simulink model "Modeling_Fix"  (R2023a)
settings: Solver=VariableStepAuto  StartTime=0.0  StopTime=40  RelTol=1e-3
undefined symbols (not defined in the file): ddx, ddy, ddz, dx, dy, dz, g, init, mass, ModelInit_AngEuler, ModelInit_PosE, ModelInit_RateB, ModelInit_VelB, ModelParam_uavJ, ModelParam_uavMass, p, pitch, q, r, roll, rotorCm, rotorCt, rotorD, ss_est_new, X, Y, yaw, Z
libraries: sharedutil x3, slident x1, slpidlib x1
settings Model: Creator=HP  LastModifiedBy=LENOVO

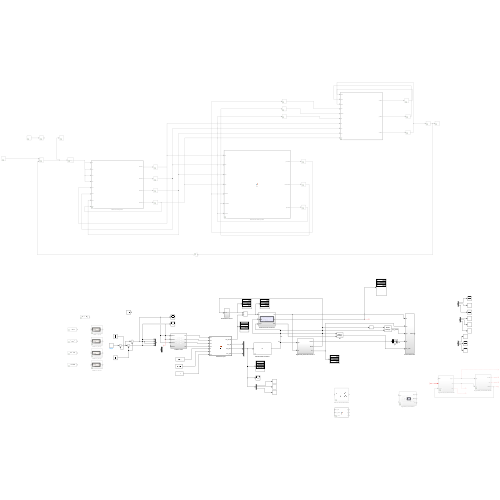
[thumbnail: Simulink's stored preview of the top-level diagram]
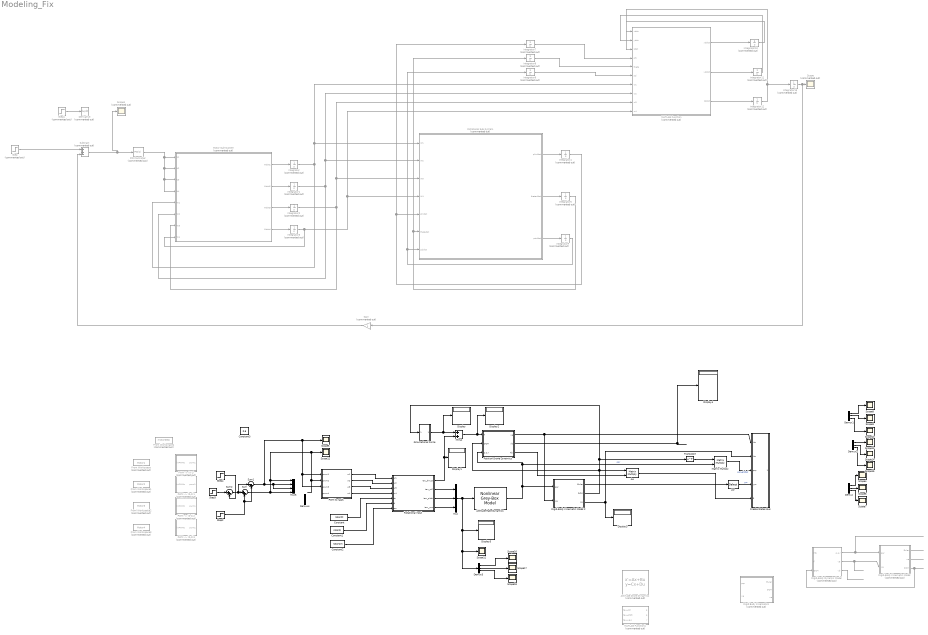
== system Modeling_Fix ==
  Ae : Product  Multiplication=Matrix(*)
  Attitude Drone Dynamics : StateSpace  Commented=on  A=ss_est_new.A  B=ss_est_new.B  C=ss_est_new.C  D=ss_est_new.D  InitialCondition=0
  Attitude Rate Dynamics : slident/Models/Nonlinear Grey-Box Model  nlsys=m  X0='m'
  Constant : Constant  Value=rotorCt
  Constant1 : Constant  Value=rotorD
  Constant2 : Constant  Value=rotorCm
  Constant3 : Constant  Value=0.6
  Create States Bus : Subsystem
  Demux{,1..3} (4 alike) : Demux  Outputs=3
  Demux4 : Demux
  Derivative : Derivative  Commented=on
  Display{,1..5} (6 alike) : Display
  From Workspace : FromWorkspace  Commented=on  VariableName=Motor1  SampleTime=0.25
  From Workspace1 : FromWorkspace  Commented=on  VariableName=Motor2  SampleTime=0.25
  From Workspace2 : FromWorkspace  Commented=on  VariableName=Motor3  SampleTime=0.25
  From Workspace3 : FromWorkspace  Commented=on  VariableName=Motor4  SampleTime=0.25
  From Workspace4 : FromWorkspace  Commented=on  VariableName=motorStep  SampleTime=0.25
  Gain : Gain  Commented=on
  Gravitational Force : Subsystem
  Integrator{,1..13} (14 alike) : Integrator  Commented=on
  MATLAB Function : MATLAB Function  Commented=on  TreatAsAtomicUnit=on
  MATLAB Function1 : MATLAB Function  Commented=on  TreatAsAtomicUnit=on
  Matrix Multiply : Product  Multiplication=Matrix(*)
  Minus : Sum
  Motor Sub-System : MATLAB Function  Commented=on  TreatAsAtomicUnit=on
  Mux : Mux  Inputs=3
  Mux5 : Mux
  PID Controller : slpidlib/PID Controller  Commented=on  Controller=PID  Form=Parallel  TimeDomain=Continuous-time  UseExternalTs=off  SampleTime=-1  IntegratorMethod=Forward Euler  FilterMethod=Forward Euler  ControllerParametersSource=internal  P=0.1  I=1  UseKiTs=off  D=0  N=100  UseFilter=on  TunerSelectOption=Transfer Function Based (PID Tuner App)  InitialConditionSource=internal  InitialConditionForIntegrator=0  InitialConditionForFilter=0  DifferentiatorICPrevScaledInput=0  ExternalReset=none  TrackingMode=off  Kt=1  LimitOutput=off  SatLimitsSource=internal  UpperSaturationLimit=inf  LowerSaturationLimit=-inf  LinearizeAsGain=on  AntiWindupMode=none  Kb=1  LimitIntegrator=off  UpperIntegratorSaturationLimit=inf  LowerIntegratorSaturationLimit=-inf  POutMin=[]  POutMax=[]  IOutMin=[]  IOutMax=[]  DOutMin=[]  DOutMax=[]  NOutMin=[]  NOutMax=[]  SumOutMin=[]  SumOutMax=[]  SaturationOutMin=[]  SaturationOutMax=[]  PParamMin=[]  PParamMax=[]  IParamMin=[]  IParamMax=[]  DParamMin=[]  DParamMax=[]  NParamMin=[]  NParamMax=[]  KbParamMin=[]  KbParamMax=[]  KtParamMin=[]  KtParamMax=[]  KbOutMin=[]  KbOutMax=[]  KtOutMin=[]  KtOutMax=[]  IntegratorOutMin=[]  IntegratorOutMax=[]  FilterOutMin=[]  FilterOutMax=[]  SumI1OutMin=[]  SumI1OutMax=[]  SumI2OutMin=[]  SumI2OutMax=[]  SumI3OutMin=[]  SumI3OutMax=[]  SumI4OutMin=[]  SumI4OutMax=[]  SumDOutMin=[]  SumDOutMax=[]  DifferentiatorOutMin=[]  DifferentiatorOutMax=[]  FilterDiffOutCoefMin=[]  FilterDiffOutCoefMax=[]  ReciprocalOutMin=[]  ReciprocalOutMax=[]  SumDenOutMin=[]  SumDenOutMax=[]  SumNumOutMin=[]  SumNumOutMax=[]  DivideOutMin=[]  DivideOutMax=[]  UdiffTsProdOutMin=[]  UdiffTsProdOutMax=[]  NTsProdOutMin=[]  NTsProdOutMax=[]  UintegralTsProdOutMin=[]  UintegralTsProdOutMax=[]  UngainTsProdOutMin=[]  UngainTsProdOutMax=[]  ClampingZeroOutDataTypeStr=Inherit: Inherit via back propagation  ClampingZeroOutMin=[]  ClampingZeroOutMax=[]  FilterDenConstantOutDataTypeStr=Inherit: Inherit via back propagation  FilterDenConstantOutMin=[]  FilterDenConstantOutMax=[]  PCopyOutDataTypeStr=Inherit: Inherit via back propagation  PCopyOutMin=[]  PCopyOutMax=[]  NCopyOutDataTypeStr=Inherit: Inherit via back propagation  NCopyOutMin=[]  NCopyOutMax=[]  IntegratorContinuousStateAttributes=''  IntegratorStateMustResolveToSignalObject=off  IntegratorRTWStateStorageClass=Auto  FilterContinuousStateAttributes=''  FilterStateMustResolveToSignalObject=off  FilterRTWStateStorageClass=Auto  ParallelPVariant=InternalParameters  IdealPVariant=Disabled  IVariant=InternalParameters  DVariant=InternalParameters  IntegratorVariant=Continuous  SatVariant=Disabled  AWVariant=Passthrough  PCopyVariant=Disabled  TRVariant=Disabled  FdbkBlocksVariant=Forward  IdealPFdbkVariant=Disabled  SatFdbkVariant=Disabled  DerivativeFilterVariant=ContFilter  NVariant=InternalParameters  NCopyVariant=Disabled  FilterICVariant=InternalICsFilter  IntegratorICVariant=InternalICs  ExternalResetVariant=Disabled  TRSumVariant=Passthrough  SumFdbkVariant=Disabled  SumVariant=Sum_PID  TsampFilterVariant=InternalTs  TsampNgainVariant=Passthrough  TsampIntegralVariant=Disabled_SignalSpec  ExternalSaturationOutDataTypeStr=Inherit: Same as second input
  "PWM -> (0-1)" : Subsystem  Commented=on
  "PWM -> (0-1)1" : Subsystem  Commented=on
  "PWM -> (0-1)2" : Subsystem  Commented=on
  "PWM -> (0-1)3" : Subsystem  Commented=on
  PWM to rad/s : Subsystem
  Position Drone Dynamics : Subsystem
  Rigid Body Kinematics : Subsystem  Commented=on
  Rigid-Body Dynamic Model : Subsystem  Commented=on
  "Rigid-Body Kinematic Model " : Subsystem  Commented=on
  Rigid-Body Kinematic Model 2 : Subsystem
  Rotational Input : MATLAB Function  TreatAsAtomicUnit=on
  Rotational Sub-System : MATLAB Function  Commented=on  TreatAsAtomicUnit=on
  Scope : Scope  Commented=on
  Scope1 : Scope  Commented=on
  Scope{4..18} (15 alike) : Scope
  Step : Step  Commented=on  Time=0  SampleTime=0
  Step1 : Step  Commented=on  Time=200  After=99  SampleTime=0
  Step2 : Step  Time=0  After=0.9  SampleTime=0.25
  Step3 : Step  Time=10  After=0.01  SampleTime=0.25
  Step4 : Step  Time=11  After=0.01  SampleTime=0.25
  Subtract : Sum  Commented=on  Inputs=++-
  Sum : Sum  Inputs=|++
  Sum1 : Sum  Inputs=|-+
  Sum2 : Sum  Inputs=|+-
  Transpose : Math  Operator=transpose
  ypr : Selector  InputPortWidth=3  IndexOptions=Index vector (dialog)  Indices=[3 2 1]  OutputSizes=1
  wires:
  Motor Sub-System/1(Wdot1) -> Integrator/1
  Integrator/1 -> MATLAB Function/7(w1), Rotational Sub-System/1(W1), Motor Sub-System/5(W1)
  Motor Sub-System/2(Wdot2) -> Integrator1/1
  Motor Sub-System/3(Wdot3) -> Integrator2/1
  Motor Sub-System/4(Wdot4) -> Integrator3/1
  Integrator1/1 -> MATLAB Function/8(w2), Rotational Sub-System/2(W2), Motor Sub-System/6(W2)
  Integrator2/1 -> MATLAB Function/9(w3), Rotational Sub-System/3(W3), Motor Sub-System/7(W3)
  Integrator3/1 -> MATLAB Function/10(w4), Rotational Sub-System/4(W4), Motor Sub-System/8(W4)
  Rotational Sub-System/1(phiddot) -> Integrator4/1
  Integrator4/1 -> Integrator7/1, Rotational Sub-System/5(phidot)
  Rotational Sub-System/2(thetaddot) -> Integrator5/1
  Integrator5/1 -> Integrator8/1, Rotational Sub-System/6(thetadot)
  Rotational Sub-System/3(psiddot) -> Integrator6/1
  Integrator6/1 -> Integrator9/1, Rotational Sub-System/7(psidot)
  Integrator7/1 -> MATLAB Function/4(phi)
  Integrator8/1 -> MATLAB Function/5(theta)
  Integrator9/1 -> MATLAB Function/6(psi)
  MATLAB Function/1(xddot) -> Integrator10/1
  Integrator10/1 -> MATLAB Function/1(xdot)
  MATLAB Function/2(yddot) -> Integrator11/1
  Integrator11/1 -> MATLAB Function/2(ydot)
  Integrator12/1 -> MATLAB Function/3(zdot), Integrator13/1
  MATLAB Function/3(zddot) -> Integrator12/1
  Step/1 -> Subtract/1
  Gain/1 -> Subtract/3
  Integrator13/1 -> Gain/1, Scope/1
  Subtract/1 -> PID Controller/1, Scope1/1
  Step1/1 -> Derivative/1
  PID Controller/1 -> Motor Sub-System/4(U4), Motor Sub-System/3(U3), Motor Sub-System/2(U2), Motor Sub-System/1(U1)
  PWM to rad/s/1(w1) -> Rotational Input/1(w1)
  PWM to rad/s/2(w2) -> Rotational Input/2(w2)
  PWM to rad/s/3(w3) -> Rotational Input/3(w3)
  PWM to rad/s/4(w4) -> Rotational Input/4(w4)
  Mux/1 -> Scope11/1, Demux3/1, Display5/1, Attitude Rate Dynamics/1
  Rotational Input/1(tau_thrust) -> Minus/2, Display1/1
  Attitude Rate Dynamics/1 -> Position Drone Dynamics/3(p,q,r), Matrix Multiply/2, Rigid-Body Kinematic Model 2/1(pqr)  "pqr"
  "Rigid-Body Kinematic Model "/3(DCM) -> Rigid-Body Dynamic Model/3(DCM)
  ? -> Rigid-Body Dynamic Model/2(f)
  Rigid-Body Dynamic Model/1("p,q,r ") -> "Rigid-Body Kinematic Model "/1(pqr)
  "Rigid-Body Kinematic Model "/2("xe ") -> ?
  Rigid-Body Dynamic Model/3("vb ") -> ?
  Rigid-Body Dynamic Model/2(ve) -> "Rigid-Body Kinematic Model "/2(ve)
  "Rigid-Body Kinematic Model "/1(Euler) -> ?
  Rotational Input/2(tau_roll) -> Mux/1
  Rotational Input/3(tau_pitch) -> Mux/2
  Rotational Input/4(tau_yaw) -> Mux/3
  Rigid-Body Kinematic Model 2/1(Euler) -> ypr/1
  Position Drone Dynamics/1(ve) -> Rigid-Body Kinematic Model 2/2(ve), Create States Bus/1(Ve)
  Position Drone Dynamics/2(vb) -> Display4/1
  Position Drone Dynamics/3(Ab) -> Ae/2
  Ae/1 -> Create States Bus/5(acc_lnav)
  Constant/1 -> Rotational Input/5(ct)
  Constant1/1 -> Rotational Input/6(d)
  Constant2/1 -> Rotational Input/7(cm)
  Rigid-Body Kinematic Model 2/2(DCM) -> Transpose/1, Gravitational Force/1(DCM), Position Drone Dynamics/2(DCM), Ae/1
  Gravitational Force/1(Out1) -> Display/1, Minus/1
  Minus/1 -> Display2/1, Position Drone Dynamics/1(f)
  Step4/1 -> Sum2/2
  Step3/1 -> Sum2/1
  Step2/1 -> Sum1/2, Sum/2
  Sum/1 -> PWM to rad/s/2(pwm2), Scope12/1, Mux5/1, Mux5/4
  Sum2/1 -> Sum1/1, Sum/1
  Demux/1 -> Scope4/1
  Demux/2 -> Scope6/1
  Demux/3 -> Scope7/1
  Demux1/2 -> Scope9/1
  Demux1/3 -> Scope10/1
  Demux1/1 -> Scope8/1
  Sum1/1 -> PWM to rad/s/3(pwm3), PWM to rad/s/1(pwm1), Scope5/1, Mux5/2, Mux5/3
  Demux2/1 -> Scope13/1
  Demux2/2 -> Scope14/1
  Demux2/3 -> Scope15/1
  Demux3/2 -> Scope17/1
  Demux3/1 -> Scope16/1
  Demux3/3 -> Scope18/1
  Rigid-Body Kinematic Model 2/3("xe ") -> Create States Bus/2(Xe), Display3/1
  ypr/1 -> Create States Bus/4(ypr)  "ypr"
  Transpose/1 -> Matrix Multiply/1
  Matrix Multiply/1 -> Create States Bus/3(pqr)  "pqr_global"

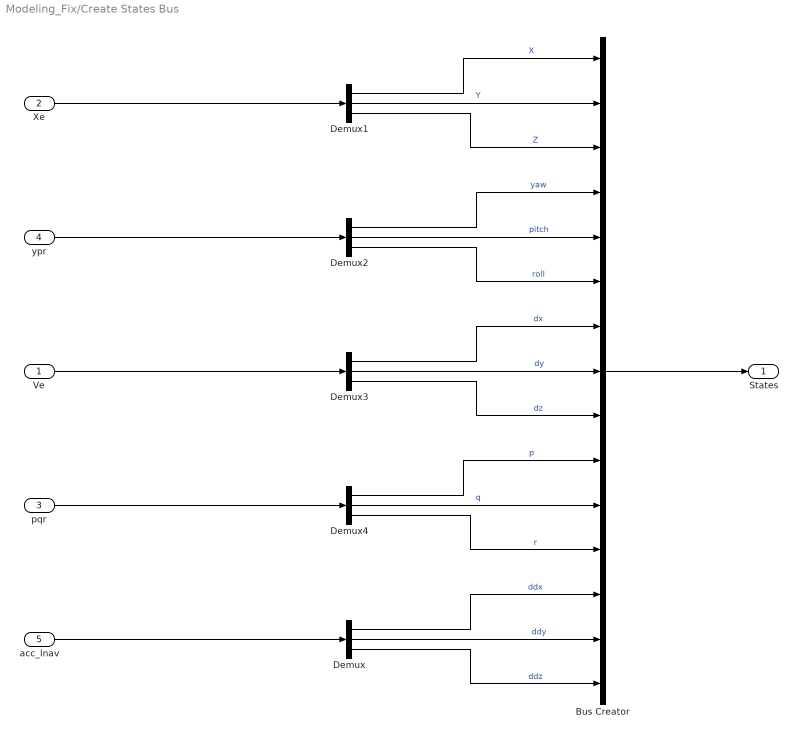
== system Modeling_Fix/Create States Bus ==
  Ve : Inport
  Xe : Inport  Port=2
  pqr : Inport  Port=3
  ypr : Inport  Port=4
  acc_lnav : Inport  Port=5
  Bus Creator : BusCreator  Inputs=X,Y,Z,yaw,pitch,roll,dx,dy,dz,p,q,r,ddx,ddy,ddz
  Demux{,1..4} (5 alike) : Demux  Outputs=3
  States : Outport
  wires:
  Demux1/1 -> Bus Creator/1  "X"
  Demux1/2 -> Bus Creator/2  "Y"
  ypr/1 -> Demux2/1
  Demux2/2 -> Bus Creator/5  "pitch"
  Demux3/2 -> Bus Creator/8  "dy"
  Demux2/3 -> Bus Creator/6  "roll"
  pqr/1 -> Demux4/1
  Ve/1 -> Demux3/1
  Demux2/1 -> Bus Creator/4  "yaw"
  Demux1/3 -> Bus Creator/3  "Z"
  Demux3/1 -> Bus Creator/7  "dx"
  Demux4/2 -> Bus Creator/11  "q"
  Demux3/3 -> Bus Creator/9  "dz"
  Demux4/3 -> Bus Creator/12  "r"
  Demux4/1 -> Bus Creator/10  "p"
  Bus Creator/1 -> States/1
  Xe/1 -> Demux1/1
  acc_lnav/1 -> Demux/1
  Demux/3 -> Bus Creator/15  "ddz"
  Demux/2 -> Bus Creator/14  "ddy"
  Demux/1 -> Bus Creator/13  "ddx"

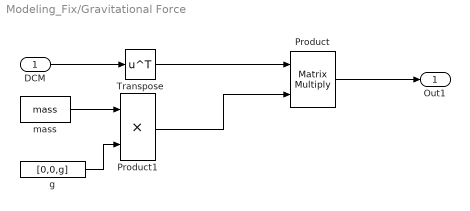
== system Modeling_Fix/Gravitational Force ==
  DCM : Inport
  Product : Product  Multiplication=Matrix(*)
  Product1 : Product
  Transpose : Math  Operator=transpose  SignedPower=on
  g : Constant  Value=[0,0,g]
  mass : Constant  Value=mass
  Out1 : Outport
  wires:
  Transpose/1 -> Product/1
  Product/1 -> Out1/1
  g/1 -> Product1/2
  mass/1 -> Product1/1
  Product1/1 -> Product/2
  DCM/1 -> Transpose/1

== system Modeling_Fix/PWM -> (0-1) ==
  note: The input is a PWM signal from 1000 to 2000,
      | which needs to be normalized to 0~1.
  inPWMs : Inport
  Constant2 : Constant  Value=900
  Gain1 : Gain  Gain=1/1100
  Saturation : Saturate  UpperLimit=1  LowerLimit=0
  Sum : Sum  Inputs=|+-
  pwm1 : Outport
  wires:
  inPWMs/1 -> Sum/1
  Constant2/1 -> Sum/2
  Gain1/1 -> Saturation/1
  Sum/1 -> Gain1/1
  Saturation/1 -> pwm1/1

== system Modeling_Fix/PWM -> (0-1)1 ==
  note: The input is a PWM signal from 1000 to 2000,
      | which needs to be normalized to 0~1.
  inPWMs : Inport
  Constant2 : Constant  Value=900
  Gain1 : Gain  Gain=1/1100
  Saturation : Saturate  UpperLimit=1  LowerLimit=0
  Sum : Sum  Inputs=|+-
  pwm1 : Outport
  wires:
  inPWMs/1 -> Sum/1
  Constant2/1 -> Sum/2
  Gain1/1 -> Saturation/1
  Sum/1 -> Gain1/1
  Saturation/1 -> pwm1/1

== system Modeling_Fix/PWM -> (0-1)2 ==
  note: The input is a PWM signal from 1000 to 2000,
      | which needs to be normalized to 0~1.
  inPWMs : Inport
  Constant2 : Constant  Value=900
  Gain1 : Gain  Gain=1/1100
  Saturation : Saturate  UpperLimit=1  LowerLimit=0
  Sum : Sum  Inputs=|+-
  pwm1 : Outport
  wires:
  inPWMs/1 -> Sum/1
  Constant2/1 -> Sum/2
  Gain1/1 -> Saturation/1
  Sum/1 -> Gain1/1
  Saturation/1 -> pwm1/1

== system Modeling_Fix/PWM -> (0-1)3 ==
  note: The input is a PWM signal from 1000 to 2000,
      | which needs to be normalized to 0~1.
  inPWMs : Inport
  Constant2 : Constant  Value=900
  Gain1 : Gain  Gain=1/1100
  Saturation : Saturate  UpperLimit=1  LowerLimit=0
  Sum : Sum  Inputs=|+-
  pwm1 : Outport
  wires:
  inPWMs/1 -> Sum/1
  Constant2/1 -> Sum/2
  Gain1/1 -> Saturation/1
  Sum/1 -> Gain1/1
  Saturation/1 -> pwm1/1

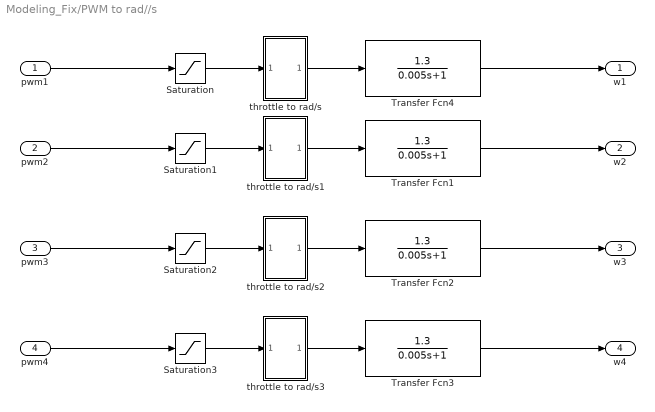
== system Modeling_Fix/PWM to rad//s ==
  pwm1 : Inport
  pwm2 : Inport  Port=2
  pwm3 : Inport  Port=3
  pwm4 : Inport  Port=4
  Saturation{,1..3} (4 alike) : Saturate  UpperLimit=1  LowerLimit=0
  Transfer Fcn{1..4} (4 alike) : TransferFcn  Numerator=1.3  Denominator=[0.005 1]
  throttle to rad/s : Subsystem
  throttle to rad/s1 : Subsystem
  throttle to rad/s2 : Subsystem
  throttle to rad/s3 : Subsystem
  w1 : Outport
  w2 : Outport  Port=2
  w3 : Outport  Port=3
  w4 : Outport  Port=4
  wires:
  pwm1/1 -> Saturation/1
  pwm2/1 -> Saturation1/1
  throttle to rad/s/1(Out1) -> Transfer Fcn4/1
  Transfer Fcn4/1 -> w1/1
  throttle to rad/s3/1(Out1) -> Transfer Fcn3/1
  Transfer Fcn1/1 -> w2/1
  throttle to rad/s2/1(Out1) -> Transfer Fcn2/1
  Transfer Fcn3/1 -> w4/1
  pwm4/1 -> Saturation3/1
  Transfer Fcn2/1 -> w3/1
  pwm3/1 -> Saturation2/1
  Saturation/1 -> throttle to rad/s/1(In2)
  Saturation1/1 -> throttle to rad/s1/1(In2)
  Saturation2/1 -> throttle to rad/s2/1(In2)
  Saturation3/1 -> throttle to rad/s3/1(In2)
  throttle to rad/s1/1(Out1) -> Transfer Fcn1/1

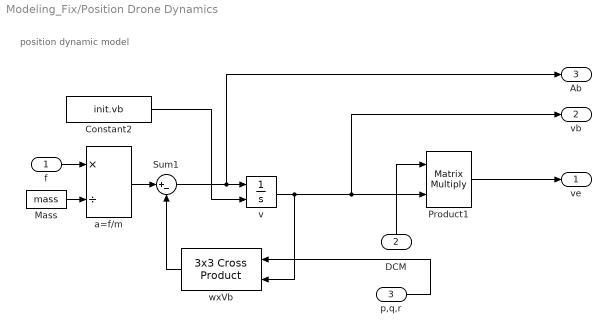
== system Modeling_Fix/Position Drone Dynamics ==
  note: position dynamic model
  f : Inport
  DCM : Inport  Port=2
  p,q,r : Inport  Port=3
  " Mass " : Constant  Value=mass
  Constant2 : Constant  Value=init.vb
  Product1 : Product  Multiplication=Matrix(*)
  Sum1 : Sum  Inputs=|+-
  a=f/m : Product  Inputs=*/
  v : Integrator  InitialConditionSource=external
  wxVb : sharedutil/3x3 Cross Product  aMode=aMode
  ve : Outport  VectorParamsAs1DForOutWhenUnconnected=off
  vb : Outport  Port=2  VectorParamsAs1DForOutWhenUnconnected=off
  Ab : Outport  Port=3
  wires:
  DCM/1 -> Product1/1
  v/1 -> vb/1, Product1/2, wxVb/2
  Sum1/1 -> Ab/1, v/1
  Constant2/1 -> v/2
  " Mass "/1 -> a=f/m/2
  wxVb/1 -> Sum1/2
  f/1 -> a=f/m/1
  p,q,r/1 -> wxVb/1
  a=f/m/1 -> Sum1/1
  Product1/1 -> ve/1

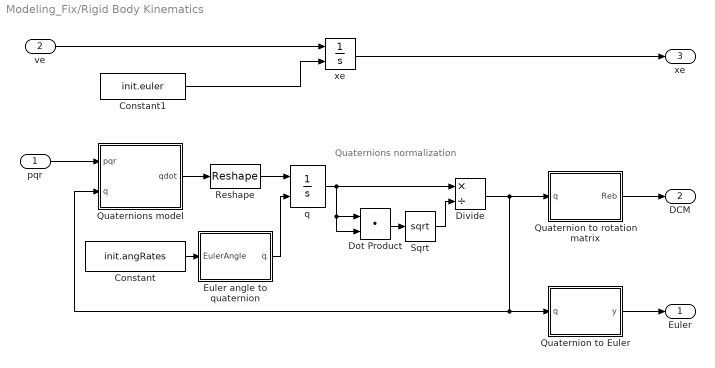
== system Modeling_Fix/Rigid Body Kinematics ==
  note: Quaternions
      | normalization
  pqr : Inport
  ve : Inport  Port=2
  Constant : Constant  Value=init.angRates
  Constant1 : Constant  Value=init.euler
  Divide : Product  Inputs=*/
  Dot Product : DotProduct  OutDataTypeStr=Inherit: Inherit via internal rule
  Euler angle to quaternion : MATLAB Function
  Quaternion to Euler : MATLAB Function
  Quaternion to rotation matrix : MATLAB Function
  Quaternions model : MATLAB Function  TreatAsAtomicUnit=on
  Reshape : Reshape  OutputDimensionality=Customize  OutputDimensions=[4,1]
  Sqrt : Sqrt
  q : Integrator  InitialConditionSource=external
  xe : Integrator  InitialConditionSource=external
  Euler : Outport  VectorParamsAs1DForOutWhenUnconnected=off
  DCM : Outport  Port=2  VectorParamsAs1DForOutWhenUnconnected=off
  "xe " : Outport  Port=3  VectorParamsAs1DForOutWhenUnconnected=off
  wires:
  q/1 -> Divide/1, Dot Product/1, Dot Product/2
  Quaternion to Euler/1(y) -> Euler/1
  Divide/1 -> Quaternion to rotation matrix/1(q), Quaternions model/2(q), Quaternion to Euler/1(q)
  Reshape/1 -> q/1
  Dot Product/1 -> Sqrt/1
  Sqrt/1 -> Divide/2
  pqr/1 -> Quaternions model/1(pqr)
  Euler angle to quaternion/1(q) -> q/2
  Quaternions model/1(qdot) -> Reshape/1
  Constant/1 -> Euler angle to quaternion/1(EulerAngle)
  Quaternion to rotation matrix/1(Reb) -> DCM/1
  Constant1/1 -> xe/2
  ve/1 -> xe/1
  xe/1 -> "xe "/1

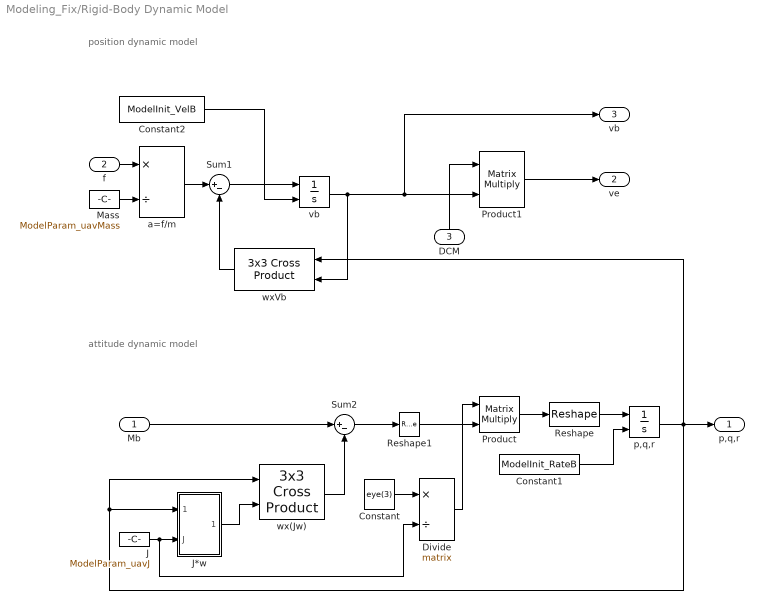
== system Modeling_Fix/Rigid-Body Dynamic Model ==
  note: attitude dynamic model
  note: position dynamic model
  Mb : Inport
  f : Inport  Port=2
  DCM : Inport  Port=3
  " Mass " : Constant  Value=ModelParam_uavMass
  Constant : Constant  Value=eye(3)
  Constant1 : Constant  Value=ModelInit_RateB
  Constant2 : Constant  Value=ModelInit_VelB
  Divide : Product  Inputs=*/  Multiplication=Matrix(*)
  "J " : Constant  Value=ModelParam_uavJ
  J*w : Subsystem
  Product : Product  Multiplication=Matrix(*)
  Product1 : Product  Multiplication=Matrix(*)
  Reshape : Reshape  OutputDimensionality=Customize  OutputDimensions=[3,1]
  Reshape1 : Reshape  OutputDimensionality=Column vector (2-D)
  Sum1 : Sum  Inputs=|+-
  Sum2 : Sum  Inputs=|+-
  a=f/m : Product  Inputs=*/
  p,q,r : Integrator  InitialConditionSource=external
  vb : Integrator  InitialConditionSource=external
  wx(Jw) : sharedutil/3x3 Cross Product  aMode=aMode
  wxVb : sharedutil/3x3 Cross Product  aMode=aMode
  "p,q,r " : Outport  VectorParamsAs1DForOutWhenUnconnected=off
  ve : Outport  Port=2  VectorParamsAs1DForOutWhenUnconnected=off
  "vb " : Outport  Port=3  VectorParamsAs1DForOutWhenUnconnected=off
  wires:
  Product/1 -> Reshape/1
  Reshape1/1 -> Product/2
  Constant/1 -> Divide/1
  Divide/1 -> Product/1
  Sum2/1 -> Reshape1/1
  "J "/1 -> Divide/2, J*w/2(J)
  p,q,r/1 -> "p,q,r "/1, J*w/1(p q r), wx(Jw)/1, wxVb/1
  J*w/1("J*w ") -> wx(Jw)/2
  Mb/1 -> Sum2/1
  wx(Jw)/1 -> Sum2/2
  Constant2/1 -> vb/2
  f/1 -> a=f/m/1
  Product1/1 -> ve/1
  wxVb/1 -> Sum1/2
  a=f/m/1 -> Sum1/1
  Sum1/1 -> vb/1
  vb/1 -> Product1/2, "vb "/1, wxVb/2
  " Mass "/1 -> a=f/m/2
  DCM/1 -> Product1/1
  Reshape/1 -> p,q,r/1
  Constant1/1 -> p,q,r/2

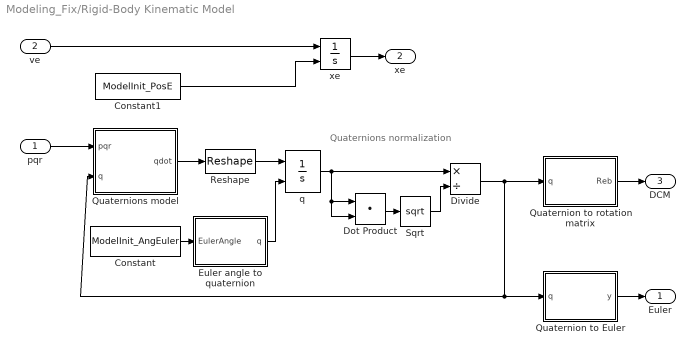
== system Modeling_Fix/Rigid-Body Kinematic Model  ==
  note: Quaternions
      | normalization
  pqr : Inport
  ve : Inport  Port=2
  Constant : Constant  Value=ModelInit_AngEuler
  Constant1 : Constant  Value=ModelInit_PosE
  Divide : Product  Inputs=*/
  Dot Product : DotProduct  OutDataTypeStr=Inherit: Inherit via internal rule
  Euler angle to quaternion : MATLAB Function
  Quaternion to Euler : MATLAB Function
  Quaternion to rotation matrix : MATLAB Function
  Quaternions model : MATLAB Function  TreatAsAtomicUnit=on
  Reshape : Reshape  OutputDimensionality=Customize  OutputDimensions=[4,1]
  Sqrt : Sqrt
  q : Integrator  InitialConditionSource=external
  xe : Integrator  InitialConditionSource=external
  Euler : Outport  VectorParamsAs1DForOutWhenUnconnected=off
  "xe " : Outport  Port=2  VectorParamsAs1DForOutWhenUnconnected=off
  DCM : Outport  Port=3  VectorParamsAs1DForOutWhenUnconnected=off
  wires:
  Divide/1 -> Quaternion to rotation matrix/1(q), Quaternions model/2(q), Quaternion to Euler/1(q)
  Dot Product/1 -> Sqrt/1
  pqr/1 -> Quaternions model/1(pqr)
  q/1 -> Divide/1, Dot Product/1, Dot Product/2
  Quaternions model/1(qdot) -> Reshape/1
  Quaternion to rotation matrix/1(Reb) -> DCM/1
  Quaternion to Euler/1(y) -> Euler/1
  Constant/1 -> Euler angle to quaternion/1(EulerAngle)
  Euler angle to quaternion/1(q) -> q/2
  Reshape/1 -> q/1
  ve/1 -> xe/1
  xe/1 -> "xe "/1
  Constant1/1 -> xe/2
  Sqrt/1 -> Divide/2

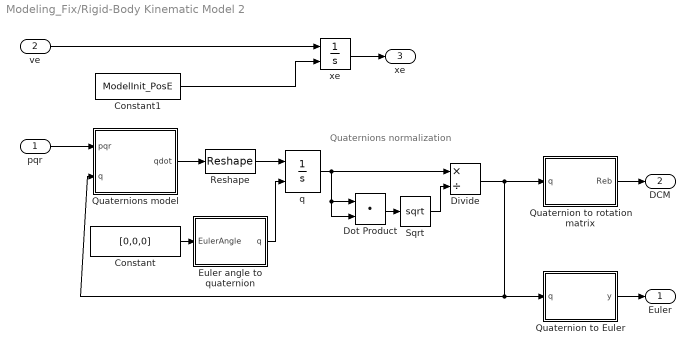
== system Modeling_Fix/Rigid-Body Kinematic Model 2 ==
  note: Quaternions
      | normalization
  pqr : Inport
  ve : Inport  Port=2
  Constant : Constant  Value=[0,0,0]
  Constant1 : Constant  Value=ModelInit_PosE
  Divide : Product  Inputs=*/
  Dot Product : DotProduct  OutDataTypeStr=Inherit: Inherit via internal rule
  Euler angle to quaternion : MATLAB Function
  Quaternion to Euler : MATLAB Function
  Quaternion to rotation matrix : MATLAB Function
  Quaternions model : MATLAB Function  TreatAsAtomicUnit=on
  Reshape : Reshape  OutputDimensionality=Customize  OutputDimensions=[4,1]
  Sqrt : Sqrt
  q : Integrator  InitialConditionSource=external
  xe : Integrator  InitialConditionSource=external
  Euler : Outport  VectorParamsAs1DForOutWhenUnconnected=off
  DCM : Outport  Port=2  VectorParamsAs1DForOutWhenUnconnected=off
  "xe " : Outport  Port=3  VectorParamsAs1DForOutWhenUnconnected=off
  wires:
  Divide/1 -> Quaternion to rotation matrix/1(q), Quaternions model/2(q), Quaternion to Euler/1(q)
  Dot Product/1 -> Sqrt/1
  pqr/1 -> Quaternions model/1(pqr)
  q/1 -> Divide/1, Dot Product/1, Dot Product/2
  Quaternions model/1(qdot) -> Reshape/1
  Quaternion to rotation matrix/1(Reb) -> DCM/1
  Quaternion to Euler/1(y) -> Euler/1
  Constant/1 -> Euler angle to quaternion/1(EulerAngle)
  Euler angle to quaternion/1(q) -> q/2
  Reshape/1 -> q/1
  ve/1 -> xe/1
  xe/1 -> "xe "/1
  Constant1/1 -> xe/2
  Sqrt/1 -> Divide/2

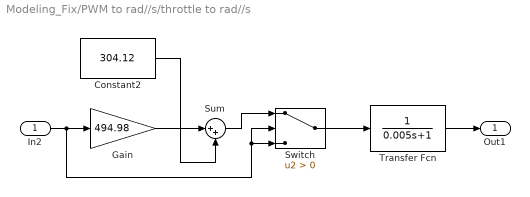
== system Modeling_Fix/PWM to rad//s/throttle to rad//s ==
  In2 : Inport
  Constant2 : Constant  Value=304.12
  Gain : Gain  Gain=494.98
  Sum : Sum  Inputs=|++
  Switch : Switch  Criteria=u2 > Threshold  SaturateOnIntegerOverflow=off  InputSameDT=off
  Transfer Fcn : TransferFcn  Denominator=[0.005 1]
  Out1 : Outport
  wires:
  Constant2/1 -> Sum/2
  Gain/1 -> Sum/1
  In2/1 -> Switch/3, Switch/2, Gain/1
  Sum/1 -> Switch/1
  Transfer Fcn/1 -> Out1/1
  Switch/1 -> Transfer Fcn/1

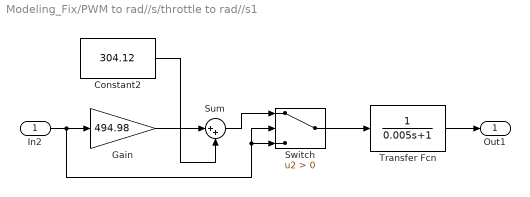
== system Modeling_Fix/PWM to rad//s/throttle to rad//s1 ==
  In2 : Inport
  Constant2 : Constant  Value=304.12
  Gain : Gain  Gain=494.98
  Sum : Sum  Inputs=|++
  Switch : Switch  Criteria=u2 > Threshold  SaturateOnIntegerOverflow=off  InputSameDT=off
  Transfer Fcn : TransferFcn  Denominator=[0.005 1]
  Out1 : Outport
  wires:
  Constant2/1 -> Sum/2
  Gain/1 -> Sum/1
  In2/1 -> Switch/3, Switch/2, Gain/1
  Sum/1 -> Switch/1
  Transfer Fcn/1 -> Out1/1
  Switch/1 -> Transfer Fcn/1

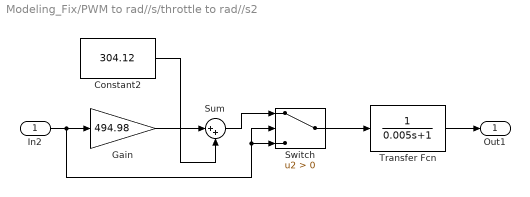
== system Modeling_Fix/PWM to rad//s/throttle to rad//s2 ==
  In2 : Inport
  Constant2 : Constant  Value=304.12
  Gain : Gain  Gain=494.98
  Sum : Sum  Inputs=|++
  Switch : Switch  Criteria=u2 > Threshold  SaturateOnIntegerOverflow=off  InputSameDT=off
  Transfer Fcn : TransferFcn  Denominator=[0.005 1]
  Out1 : Outport
  wires:
  Constant2/1 -> Sum/2
  Gain/1 -> Sum/1
  In2/1 -> Switch/3, Switch/2, Gain/1
  Sum/1 -> Switch/1
  Transfer Fcn/1 -> Out1/1
  Switch/1 -> Transfer Fcn/1

== system Modeling_Fix/PWM to rad//s/throttle to rad//s3 ==
  In2 : Inport
  Constant2 : Constant  Value=304.12
  Gain : Gain  Gain=494.98
  Sum : Sum  Inputs=|++
  Switch : Switch  Criteria=u2 > Threshold  SaturateOnIntegerOverflow=off  InputSameDT=off
  Transfer Fcn : TransferFcn  Denominator=[0.005 1]
  Out1 : Outport
  wires:
  Constant2/1 -> Sum/2
  Gain/1 -> Sum/1
  In2/1 -> Switch/3, Switch/2, Gain/1
  Sum/1 -> Switch/1
  Transfer Fcn/1 -> Out1/1
  Switch/1 -> Transfer Fcn/1

== system Modeling_Fix/Rigid-Body Dynamic Model/J*w ==
  p q r : Inport
  J : Inport  Port=2
  J*w : Product  Multiplication=Matrix(*)
  "J*w " : Outport  VectorParamsAs1DForOutWhenUnconnected=off
  wires:
  J*w/1 -> "J*w "/1
  J/1 -> J*w/1
  p q r/1 -> J*w/2

== matlab function Modeling_Fix/Rigid-Body Kinematic Model /Quaternion to rotation matrix ==
  data: q input; Reb output
function Reb = fcn(q)
%Function description;
%  The rotation matrix of the Aircraft-Body Coordinate Frame (ABCF) to the
%  Earth-Fixed Coordinate Frame (EFCF) is obtained from the quaternions
Reb = [q(1)*q(1) + q(2)*q(2) - q(3)*q(3) - q(4)*q(4), 2*(q(2)*q(3) - q(1)*q(4)), 2*(q(2)*q(4) + q(1)*q(3))
           2*(q(2)*q(3) + q(1)*q(4)), q(1)*q(1) - q(2)*q(2) + q(3)*q(3) - q(4)*q(4), 2*(q(3)*q(4) - q(1)*q(2))
           2*(q(2)*q(4) - q(1)*q(3)), 2*(q(3)*q(4) + q(1)*q(2)), q(1)*q(1) - q(2)*q(2) - q(3)*q(3) + q(4)*q(4)];

== matlab function Modeling_Fix/Rigid-Body Kinematic Model /Quaternion to Euler ==
  data: q input; y output
function y = fcn(q)
 %Function description:
%  Quaternions to Euler
phi = atan2(2*(q(1)*q(2) + q(3)*q(4)), (1 - 2*(q(2)*q(2) + q(3)*q(3))));
theta = asin(2*(q(1)*q(3) - q(2)*q(4)));
psi = atan2(2*(q(1)*q(4) + q(2)*q(3)), (1 - 2*(q(3)*q(3) + q(4)*q(4))));
y = [phi theta psi];

== matlab function Modeling_Fix/Rigid-Body Kinematic Model /Quaternions model ==
  data: pqr input; qdot output; q input
function qdot = fcn(pqr, q)
%Function description:
%  Quaternions model
qdot = 0.5*[0, -pqr(1), -pqr(2), -pqr(3); pqr(1), 0, pqr(3), -pqr(2); pqr(2), -pqr(3), 0, pqr(1); pqr(3), pqr(2), -pqr(1), 0]*q;

== matlab function Modeling_Fix/Rigid-Body Kinematic Model /Euler angle to quaternion ==
  data: EulerAngle input; q output
function q = fcn(EulerAngle)
%Function description:
%  Get quaternions from Euler angle
q0 =  cos(EulerAngle(1)/2)*cos(EulerAngle(2)/2)*cos(EulerAngle(3)/2) + sin(EulerAngle(1)/2)*sin((EulerAngle(2)/2))*sin((EulerAngle(3)/2));
q1 = sin(EulerAngle(1)/2)*cos(EulerAngle(2)/2)*cos(EulerAngle(3)/2) - cos(EulerAngle(1)/2)*sin((EulerAngle(2)/2))*sin((EulerAngle(3)/2));
q2 = cos(EulerAngle(1)/2)*sin(EulerAngle(2)/2)*cos(EulerAngle(3)/2) + sin(EulerAngle(1)/2)*cos((EulerAngle(2)/2))*sin((EulerAngle(3)/2));
q3 = cos(EulerAngle(1)/2)*cos(EulerAngle(2)/2)*sin(EulerAngle(3)/2) - sin(EulerAngle(1)/2)*sin((EulerAngle(2)/2))*cos((EulerAngle(3)/2));
q = [q0 q1 q2 q3]';

== matlab function Modeling_Fix/Rigid Body Kinematics/Quaternion to Euler ==
  data: q input; y output
function y = fcn(q)
 %Function description:
%  Quaternions to Euler
phi = atan2(2*(q(1)*q(2) + q(3)*q(4)), (1 - 2*(q(2)*q(2) + q(3)*q(3))));
theta = asin(2*(q(1)*q(3) - q(2)*q(4)));
psi = atan2(2*(q(1)*q(4) + q(2)*q(3)), (1 - 2*(q(3)*q(3) + q(4)*q(4))));
y = [phi theta psi];

== matlab function Modeling_Fix/Rigid Body Kinematics/Quaternion to rotation matrix ==
  data: q input; Reb output
function Reb = fcn(q)
%Function description;
%  The rotation matrix of the Aircraft-Body Coordinate Frame (ABCF) to the
%  Earth-Fixed Coordinate Frame (EFCF) is obtained from the quaternions
Reb = [q(1)*q(1) + q(2)*q(2) - q(3)*q(3) - q(4)*q(4), 2*(q(2)*q(3) - q(1)*q(4)), 2*(q(2)*q(4) + q(1)*q(3))
           2*(q(2)*q(3) + q(1)*q(4)), q(1)*q(1) - q(2)*q(2) + q(3)*q(3) - q(4)*q(4), 2*(q(3)*q(4) - q(1)*q(2))
           2*(q(2)*q(4) - q(1)*q(3)), 2*(q(3)*q(4) + q(1)*q(2)), q(1)*q(1) - q(2)*q(2) - q(3)*q(3) + q(4)*q(4)];

== matlab function Modeling_Fix/Rigid Body Kinematics/Quaternions model ==
  data: pqr input; qdot output; q input
function qdot = fcn(pqr, q)
%Function description:
%  Quaternions model
qdot = 0.5*[0, -pqr(1), -pqr(2), -pqr(3); pqr(1), 0, pqr(3), -pqr(2); pqr(2), -pqr(3), 0, pqr(1); pqr(3), pqr(2), -pqr(1), 0]*q;

== matlab function Modeling_Fix/Rigid-Body Kinematic Model 2/Euler angle to quaternion ==
  data: EulerAngle input; q output
function q = fcn(EulerAngle)
%Function description:
%  Get quaternions from Euler angle
q0 =  cos(EulerAngle(1)/2)*cos(EulerAngle(2)/2)*cos(EulerAngle(3)/2) + sin(EulerAngle(1)/2)*sin((EulerAngle(2)/2))*sin((EulerAngle(3)/2));
q1 = sin(EulerAngle(1)/2)*cos(EulerAngle(2)/2)*cos(EulerAngle(3)/2) - cos(EulerAngle(1)/2)*sin((EulerAngle(2)/2))*sin((EulerAngle(3)/2));
q2 = cos(EulerAngle(1)/2)*sin(EulerAngle(2)/2)*cos(EulerAngle(3)/2) + sin(EulerAngle(1)/2)*cos((EulerAngle(2)/2))*sin((EulerAngle(3)/2));
q3 = cos(EulerAngle(1)/2)*cos(EulerAngle(2)/2)*sin(EulerAngle(3)/2) - sin(EulerAngle(1)/2)*sin((EulerAngle(2)/2))*cos((EulerAngle(3)/2));
q = [q0 q1 q2 q3]';

== matlab function Modeling_Fix/Rigid-Body Kinematic Model 2/Quaternion to Euler ==
  data: q input; y output
function y = fcn(q)
 %Function description:
%  Quaternions to Euler
phi = atan2(2*(q(1)*q(2) + q(3)*q(4)), (1 - 2*(q(2)*q(2) + q(3)*q(3))));
theta = asin(2*(q(1)*q(3) - q(2)*q(4)));
psi = atan2(2*(q(1)*q(4) + q(2)*q(3)), (1 - 2*(q(3)*q(3) + q(4)*q(4))));
y = [phi theta psi];

== matlab function Modeling_Fix/Rigid-Body Kinematic Model 2/Quaternion to rotation matrix ==
  data: q input; Reb output
function Reb = fcn(q)
%Function description;
%  The rotation matrix of the Aircraft-Body Coordinate Frame (ABCF) to the
%  Earth-Fixed Coordinate Frame (EFCF) is obtained from the quaternions
Reb = [q(1)*q(1) + q(2)*q(2) - q(3)*q(3) - q(4)*q(4), 2*(q(2)*q(3) - q(1)*q(4)), 2*(q(2)*q(4) + q(1)*q(3))
           2*(q(2)*q(3) + q(1)*q(4)), q(1)*q(1) - q(2)*q(2) + q(3)*q(3) - q(4)*q(4), 2*(q(3)*q(4) - q(1)*q(2))
           2*(q(2)*q(4) - q(1)*q(3)), 2*(q(3)*q(4) + q(1)*q(2)), q(1)*q(1) - q(2)*q(2) - q(3)*q(3) + q(4)*q(4)];

== matlab function Modeling_Fix/Rigid-Body Kinematic Model 2/Quaternions model ==
  data: pqr input; qdot output; q input
function qdot = fcn(pqr, q)
%Function description:
%  Quaternions model
qdot = 0.5*[0, -pqr(1), -pqr(2), -pqr(3); pqr(1), 0, pqr(3), -pqr(2); pqr(2), -pqr(3), 0, pqr(1); pqr(3), pqr(2), -pqr(1), 0]*q;

== matlab function Modeling_Fix/Rotational Sub-System ==
  data: W1 input; phiddot output; W2 input; W3 input; W4 input; phidot input; thetadot input; psidot input; thetaddot output; psiddot output
function [phiddot, thetaddot, psiddot] = fcn(W1,W2,W3,W4,phidot,thetadot,psidot)
Ixx = 1;
Iyy = 1;
Izz = 1;
l = 1;
alpha = 1; 
beta = 1;
Ca = 1;
CT = 1;
rho = 1;
A = 1;
r =1;

phiddot = ((Iyy - Izz)*(thetadot*psidot) + (W1^2 - W2^2 - W3^2 + W4^2)*0.5*l*sin(alpha)*Ca*rho*A*r^2)/Ixx;
thetaddot = ((Izz - Ixx)*(phidot*psidot) + (W1^2 + W2^2 - W3^2 - W4^2)*0.5*l*sin(beta)*Ca*rho*A*r^2)/Iyy;
psiddot = ((Ixx - Iyy)*(phidot*thetadot) + (-W1^2 + W2^2 - W3^2 + W4^2)*CT*rho*A*r^3)/Izz;

== matlab function Modeling_Fix/Motor Sub-System ==
  data: U1 input; U2 input; U3 input; U4 input; Wdot1 output; Wdot2 output; Wdot3 output; Wdot4 output; W1 input; W2 input; W3 input; W4 input
function [Wdot1,Wdot2,Wdot3,Wdot4] = fcn(U1,U2,U3,U4,W1,W2,W3,W4)
Ke = 1;
Ktm = 1;
Rm =  1;
Jm = 1;
d = 1;
Wo = 1.56524;
n = 1;
r_g = 1;
dm = 1;
A = -(((Ke*Ktm)/(Rm*Jm)) + ((2*d*Wo)/(n*r_g^3*Jm)));
B = Ktm/(Rm*Jm);
C = (dm*Wo^2)/(n*r_g^3*Jm);
Wdot1 = A*W1 + B*U1 + C ;
Wdot2 = A*W2 + B*U2 + C ;
Wdot3 = A*W3 + B*U3 + C ;
Wdot4 = A*W4 + B*U4 + C ;

== matlab function Modeling_Fix/MATLAB Function ==
  data: xdot input; xddot output; ydot input; zdot input; phi input; theta input; psi input; w1 input; w2 input; w3 input; w4 input; yddot output; zddot output
function [xddot,yddot,zddot]= fcn(xdot,ydot,zdot,phi,theta,psi,w1,w2,w3,w4)
Cx = 1;
Cy = 1;
Cz = 1;
Ca = 1;
Ac = 1;
rho = 1;
r = 1;
A = 1;
m = 1;
g = 9.8;

ax = -0.5*Cx*Ac*rho;
ay = -0.5*Cy*Ac*rho;
az = -0.5*Cz*Ac*rho;
wnew = (w1^2+w2^2+w3^2+w4^2);
Ux = (-cos(phi)*sin(theta)*cos(psi)-sin(phi)*sin(psi))*Ca*rho*A*r^2*wnew;
Uy = (-cos(phi)*sin(theta)*cos(psi)+sin(phi)*sin(psi))*Ca*rho*A*r^2*wnew;
Uz = -(cos(phi)*cos(theta))*Ca*rho *A*r^2*wnew;
xddot = (ax*xdot*abs(xdot)+Ux)/m;
yddot = (ay*ydot*abs(ydot)+Uy)/m;
zddot = (az*zdot*abs(zdot)+m*g+Uz)/m;

== matlab function Modeling_Fix/Rotational Input ==
  data: w1 input; tau_thrust output; w2 input; w3 input; w4 input; tau_roll output; tau_pitch output; tau_yaw output; ct input; d input; cm input
function [tau_thrust,tau_roll,tau_pitch,tau_yaw] = fcn(w1,w2,w3,w4,ct,d,cm)
%  quadrotor is as follows:
% 3↓   1↑
%   \ /
%   / \
% 2↑   4↓
%↑ stands for counterclockwise and ↓stands for clockwise.
% Parameters
% ct : konstanta thrust
% d : jarak properller ke CoM
% cm : konstanta momen

% M_rctcm = [-sin(pi/4)*d*ct, sin(pi/4)*d*ct, sin(pi/4)*d*ct, -sin(pi/4)*d*ct;
%         sin(pi/4)*d*ct, -sin(pi/4)*d*ct, sin(pi/4)*d*ct, -sin(pi/4)*d*ct;
%         cm, cm, -cm, -cm];
% M = M_rctcm*([w1^2;w2^2;w3^2;w4^2]);
% tau_roll = M(1);
% tau_pitch = M(2);
% tau_yaw = M(3);

tau_thrust = [0;0;-ct*(w1^2+w2^2+w3^2+w4^2)];
tau_roll = (sin(pi/4))*d*ct*(-w1^2+w2^2+w3^2-w4^2);
tau_pitch = (sin(pi/4))*d*ct*(w1^2-w2^2+w3^2-w4^2);
tau_yaw = cm*(w1^2+w2^2-w3^2-w4^2);

== matlab function Modeling_Fix/MATLAB Function1 ==
  data: tau_roll input; p output; tau_pitch input; tau_yaw input; q output; r output
function [p,q,r] = fcn(tau_roll,tau_pitch,tau_yaw)

== matlab function Modeling_Fix/Rigid Body Kinematics/Euler angle to quaternion ==
  data: EulerAngle input; q output
function q = fcn(EulerAngle)
%Function description:
%  Get quaternions from Euler angle
q0 =  cos(EulerAngle(1)/2)*cos(EulerAngle(2)/2)*cos(EulerAngle(3)/2) + sin(EulerAngle(1)/2)*sin((EulerAngle(2)/2))*sin((EulerAngle(3)/2));
q1 = sin(EulerAngle(1)/2)*cos(EulerAngle(2)/2)*cos(EulerAngle(3)/2) - cos(EulerAngle(1)/2)*sin((EulerAngle(2)/2))*sin((EulerAngle(3)/2));
q2 = cos(EulerAngle(1)/2)*sin(EulerAngle(2)/2)*cos(EulerAngle(3)/2) + sin(EulerAngle(1)/2)*cos((EulerAngle(2)/2))*sin((EulerAngle(3)/2));
q3 = cos(EulerAngle(1)/2)*cos(EulerAngle(2)/2)*sin(EulerAngle(3)/2) - sin(EulerAngle(1)/2)*sin((EulerAngle(2)/2))*cos((EulerAngle(3)/2));
q = [q0 q1 q2 q3]';
